simulink model "que4"  (R2020b)
settings: Solver=VariableStepAuto  StartTime=0.0  StopTime=10.0  RelTol=1e-3
settings Model: Creator=ANUJA  LastModifiedBy=ANUJA

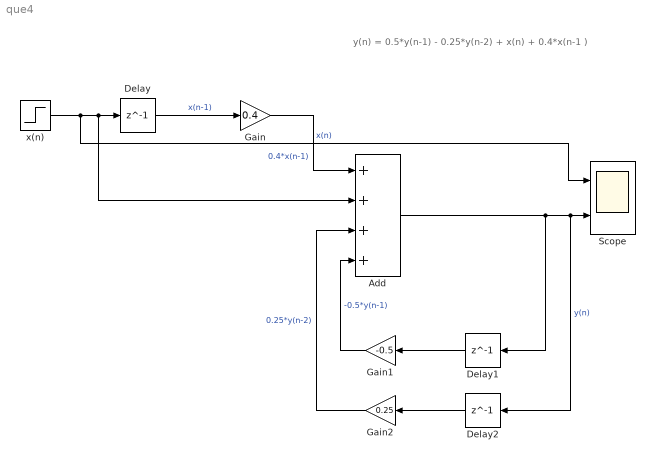
== system que4 ==
  note: y(n) = 0.5*y(n-1) - 0.25*y(n-2) + x(n) + 0.4*x(n-1 )
  Add : Sum  Inputs=++++
  Delay : Delay  DelayLength=1  InitialCondition=0
  Delay1 : Delay  DelayLength=1  InitialCondition=0
  Delay2 : Delay  DelayLength=1  InitialCondition=0
  Gain : Gain  Gain=0.4
  Gain1 : Gain  Gain=-0.5
  Gain2 : Gain  Gain=0.25
  Scope : Scope  NumInputPorts=2
  x(n) : Step  SampleTime=0
  wires:
  x(n)/1 -> Scope/1, Add/2, Delay/1  "x(n)"
  Delay/1 -> Gain/1  "x(n-1)"
  Gain/1 -> Add/1  "0.4*x(n-1)"
  Add/1 -> Delay1/1, Delay2/1, Scope/2  "y(n)"
  Delay1/1 -> Gain1/1
  Gain1/1 -> Add/4  "-0.5*y(n-1)"
  Gain2/1 -> Add/3  "0.25*y(n-2)"
  Delay2/1 -> Gain2/1
